simulink model "controller_sdfp_host"  (Simulink 7.3)
settings: Solver=ode45  StartTime=0.0  StopTime=2  RelTol=1e-3
values from neighbouring files (symbols this model uses):
  d = 16    [one_bit_control.m]
  fixpt_adder_in_bitwidth = w    (= 24)    [one_bit_control.m]
  fixpt_adder_in_position = d    (= 16)    [one_bit_control.m]
  fixpt_adder_out_bitwidth = w    (= 24)    [one_bit_control.m]
  fixpt_adder_out_position = d    (= 16)    [one_bit_control.m]
  fixpt_gain_bitwidth = w    (= 24)    [one_bit_control.m]
  fixpt_gain_position = d    (= 16)    [one_bit_control.m]
  k = 2^k_bitshift    (= 0.0001220703125)    [one_bit_control.m]
  p0 = (109.9*Ki)*T^3*k^-3    [one_bit_control.m]
  p1 = (20.78*Ki+109.9*Kp)*T^2*k^-2    [one_bit_control.m]
  p2 = (Ki+20.78*Kp)*T*k^-1    [one_bit_control.m]
  p3 = Kp    (= 8)    [one_bit_control.m]
  q0 = 0*T^3*k^-3    [one_bit_control.m]
  q1 = 174.8*T^2*k^-2    [one_bit_control.m]
  q2 = 26.33*T*k^-1    [one_bit_control.m]
  T = ts    [one_bit_control.m]
  ts = 1/Fs    [one_bit_control.m]
  ts_k_gain1 = k_bitshift - Fs_power_2    [one_bit_control.m]
  ts_k_gain2 = k_bitshift - Fs_power_2    [one_bit_control.m]
  ts_k_gain3 = k_bitshift - Fs_power_2    [one_bit_control.m]
  w = 24    [one_bit_control.m]
libraries: simulink x16, cstblocks x5, commnoisgen2 x1, simulink_extras x1
(part 2 of 2)

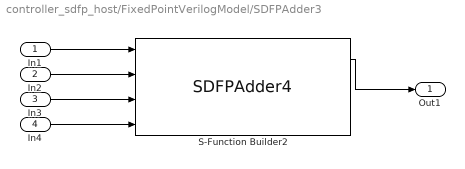
== system controller_sdfp_host/FixedPointVerilogModel/SDFPAdder3 ==
  In1 : Inport  OutDataType=fixdt(1, 16)  OutScaling=2^0
  In2 : Inport  Port=2  OutDataType=fixdt(1, 16)  OutScaling=2^0
  In3 : Inport  Port=3  OutDataType=fixdt(1, 16)  OutScaling=2^0
  In4 : Inport  Port=4  OutDataType=fixdt(1, 16)  OutScaling=2^0
  S-Function Builder2 : S-Function  InitFcn=try, set_param(gcb,'FunctionName','SDFPAdder4'), end  FunctionName=SDFPAdder4  Parameters=uint32(in_bitwidth),uint32(in_fp_position),uint32(out_bitwidth),uint32(out_fp_position)  SFunctionModules=SDFPAdder4_wrapper  WizardData=DataTag17  EnableBusSupport=off  mask(S-Function Builder){}
      mask help: The S-Function Builder block creates a wrapper C-MEX S-function from your supplied C code with multiple input ports, output ports, and a variable number of scalar, vector, or matrix parameters. The input and output ports can propagate Simulink built-in data types, fixed-point datatypes, complex, frame, 1-D, and 2-D signals. This block also supports discrete and continuous states of type real. You can optionally have the block generate a TLC file to be used with Real-Time Workshop for code generation.
      mask init: same as controller_sdfp_host/FixedPointVerilogModel/FloatForScope1/S-Function Builder
      settings: CopyFcn=set_param(gcbh,'LinkStatus','none')  PreSaveFcn=try, set_param(gcb,'FunctionName','SDFPAdder4'), end  OpenFcn=sfunctionwizard(gcbh)
      mask Display: plot(val(:,1),val(:,2)),disp(sys)port_label('input',1,'in0')port_label('input',2,'in1')port_label('input',3,'in2')port_label('input',4,'in3')port_label('output',1,'adder_out')
  Out1 : Outport  OutDataType=fixdt(1, 16)  OutScaling=2^0
  wires:
  In1/1 -> S-Function Builder2/1
  In2/1 -> S-Function Builder2/2
  In3/1 -> S-Function Builder2/3
  In4/1 -> S-Function Builder2/4
  S-Function Builder2/1 -> Out1/1

== system controller_sdfp_host/FixedPointVerilogModel/SDFPAdder4 ==
  In1 : Inport  OutDataType=fixdt(1, 16)  OutScaling=2^0
  In2 : Inport  Port=2  OutDataType=fixdt(1, 16)  OutScaling=2^0
  In3 : Inport  Port=3  OutDataType=fixdt(1, 16)  OutScaling=2^0
  In4 : Inport  Port=4  OutDataType=fixdt(1, 16)  OutScaling=2^0
  S-Function Builder2 : S-Function  InitFcn=try, set_param(gcb,'FunctionName','SDFPAdder4'), end  FunctionName=SDFPAdder4  Parameters=uint32(in_bitwidth),uint32(in_fp_position),uint32(out_bitwidth),uint32(out_fp_position)  SFunctionModules=SDFPAdder4_wrapper  WizardData=DataTag18  EnableBusSupport=off  mask(S-Function Builder){}
      mask help: The S-Function Builder block creates a wrapper C-MEX S-function from your supplied C code with multiple input ports, output ports, and a variable number of scalar, vector, or matrix parameters. The input and output ports can propagate Simulink built-in data types, fixed-point datatypes, complex, frame, 1-D, and 2-D signals. This block also supports discrete and continuous states of type real. You can optionally have the block generate a TLC file to be used with Real-Time Workshop for code generation.
      mask init: same as controller_sdfp_host/FixedPointVerilogModel/FloatForScope1/S-Function Builder
      settings: CopyFcn=set_param(gcbh,'LinkStatus','none')  PreSaveFcn=try, set_param(gcb,'FunctionName','SDFPAdder4'), end  OpenFcn=sfunctionwizard(gcbh)
      mask Display: plot(val(:,1),val(:,2)),disp(sys)port_label('input',1,'in0')port_label('input',2,'in1')port_label('input',3,'in2')port_label('input',4,'in3')port_label('output',1,'adder_out')
  Out1 : Outport  OutDataType=fixdt(1, 16)  OutScaling=2^0
  wires:
  In1/1 -> S-Function Builder2/1
  In2/1 -> S-Function Builder2/2
  In3/1 -> S-Function Builder2/3
  In4/1 -> S-Function Builder2/4
  S-Function Builder2/1 -> Out1/1

== system controller_sdfp_host/FixedPointVerilogModel/SDFPFromFixed ==
  In1 : Inport  OutDataType=fixdt(1, 16)  OutScaling=2^0
  S-Function Builder : S-Function  InitFcn=try, set_param(gcb,'FunctionName','SDFPFromFixed'), end  FunctionName=SDFPFromFixed  Parameters=uint32(bitwidth),uint32(fp_position)  SFunctionModules=SDFPFromFixed_wrapper fpconv  WizardData=DataTag19  EnableBusSupport=off  mask(S-Function Builder){}
      mask help: The S-Function Builder block creates a wrapper C-MEX S-function from your supplied C code with multiple input ports, output ports, and a variable number of scalar, vector, or matrix parameters. The input and output ports can propagate Simulink built-in data types, fixed-point datatypes, complex, frame, 1-D, and 2-D signals. This block also supports discrete and continuous states of type real. You can optionally have the block generate a TLC file to be used with Real-Time Workshop for code generation.
      mask init: same as controller_sdfp_host/FixedPointVerilogModel/FloatForScope1/S-Function Builder
      settings: CopyFcn=set_param(gcbh,'LinkStatus','none')  PreSaveFcn=try, set_param(gcb,'FunctionName','SDFPFromFixed'), end  OpenFcn=sfunctionwizard(gcbh)
      mask Display: plot(val(:,1),val(:,2)),disp(sys)port_label('input',1,'fixed_in')port_label('output',1,'float_out')
  Out1 : Outport  OutDataType=fixdt(1, 16)  OutScaling=2^0
  wires:
  In1/1 -> S-Function Builder/1
  S-Function Builder/1 -> Out1/1

== system controller_sdfp_host/FixedPointVerilogModel/SDFPShifter ==
  In1 : Inport  OutDataType=fixdt(1, 16)  OutScaling=2^0
  S-Function Builder3 : S-Function  InitFcn=try, set_param(gcb,'FunctionName','SDFPShifter'), end  FunctionName=SDFPShifter  Parameters=int32(shift_amount)  SFunctionModules=SDFPShifter_wrapper  WizardData=DataTag20  EnableBusSupport=off  mask(S-Function Builder){}
      mask help: The S-Function Builder block creates a wrapper C-MEX S-function from your supplied C code with multiple input ports, output ports, and a variable number of scalar, vector, or matrix parameters. The input and output ports can propagate Simulink built-in data types, fixed-point datatypes, complex, frame, 1-D, and 2-D signals. This block also supports discrete and continuous states of type real. You can optionally have the block generate a TLC file to be used with Real-Time Workshop for code generation.
      mask init: same as controller_sdfp_host/FixedPointVerilogModel/FloatForScope1/S-Function Builder
      settings: CopyFcn=set_param(gcbh,'LinkStatus','none')  PreSaveFcn=try, set_param(gcb,'FunctionName','SDFPShifter'), end  OpenFcn=sfunctionwizard(gcbh)
      mask Display: plot(val(:,1),val(:,2)),disp(sys)port_label('input',1,'sg_in')port_label('output',1,'shifter_out')
  Out1 : Outport  OutDataType=fixdt(1, 16)  OutScaling=2^0
  wires:
  In1/1 -> S-Function Builder3/1
  S-Function Builder3/1 -> Out1/1

== system controller_sdfp_host/FixedPointVerilogModel/SDFPToFixed ==
  In1 : Inport  OutDataType=fixdt(1, 16)  OutScaling=2^0
  S-Function Builder : S-Function  InitFcn=try, set_param(gcb,'FunctionName','SDFPToFixed'), end  FunctionName=SDFPToFixed  Parameters=uint32(bitwidth),uint32(fp_position)  SFunctionModules=SDFPToFixed_wrapper fpconv  WizardData=DataTag21  EnableBusSupport=off  mask(S-Function Builder){}
      mask help: The S-Function Builder block creates a wrapper C-MEX S-function from your supplied C code with multiple input ports, output ports, and a variable number of scalar, vector, or matrix parameters. The input and output ports can propagate Simulink built-in data types, fixed-point datatypes, complex, frame, 1-D, and 2-D signals. This block also supports discrete and continuous states of type real. You can optionally have the block generate a TLC file to be used with Real-Time Workshop for code generation.
      mask init: same as controller_sdfp_host/FixedPointVerilogModel/FloatForScope1/S-Function Builder
      settings: CopyFcn=set_param(gcbh,'LinkStatus','none')  PreSaveFcn=try, set_param(gcb,'FunctionName','SDFPToFixed'), end  OpenFcn=sfunctionwizard(gcbh)
      mask Display: plot(val(:,1),val(:,2)),disp(sys)port_label('input',1,'float_in')port_label('output',1,'fixed_out')
  Out1 : Outport  OutDataType=fixdt(1, 16)  OutScaling=2^0
  wires:
  In1/1 -> S-Function Builder/1
  S-Function Builder/1 -> Out1/1

== system controller_sdfp_host/FixedPointVerilogModel/Subsystem ==
  In1 : Inport  OutDataType=fixdt(1, 16)  OutScaling=2^0
  S-Function Builder : S-Function  InitFcn=try, set_param(gcb,'FunctionName','SDFPGainSwitch'), end  FunctionName=SDFPGainSwitch  Parameters=single(gain),uint32(bitwidth),uint32(fp_position)  SFunctionModules=SDFPGainSwitch_wrapper fpconv  WizardData=DataTag22  EnableBusSupport=off  mask(S-Function Builder){}
      mask help: The S-Function Builder block creates a wrapper C-MEX S-function from your supplied C code with multiple input ports, output ports, and a variable number of scalar, vector, or matrix parameters. The input and output ports can propagate Simulink built-in data types, fixed-point datatypes, complex, frame, 1-D, and 2-D signals. This block also supports discrete and continuous states of type real. You can optionally have the block generate a TLC file to be used with Real-Time Workshop for code generation.
      mask init: same as controller_sdfp_host/FixedPointVerilogModel/FloatForScope1/S-Function Builder
      settings: CopyFcn=set_param(gcbh,'LinkStatus','none')  PreSaveFcn=try, set_param(gcb,'FunctionName','SDFPGainSwitch'), end  OpenFcn=sfunctionwizard(gcbh)
      mask Display: plot(val(:,1),val(:,2)),disp(sys)port_label('input',1,'sd_in')port_label('output',1,'gain_out')
  Out1 : Outport  OutDataType=fixdt(1, 16)  OutScaling=2^0
  wires:
  S-Function Builder/1 -> Out1/1
  In1/1 -> S-Function Builder/1

== system controller_sdfp_host/FixedPointVerilogModel/ts_and_k_gain1 ==
  In1 : Inport  OutDataType=fixdt(1, 16)  OutScaling=2^0
  S-Function Builder3 : S-Function  InitFcn=try, set_param(gcb,'FunctionName','SDFPShifter'), end  FunctionName=SDFPShifter  Parameters=int32(shift_amount)  SFunctionModules=SDFPShifter_wrapper  WizardData=DataTag23  EnableBusSupport=off  mask(S-Function Builder){}
      mask help: The S-Function Builder block creates a wrapper C-MEX S-function from your supplied C code with multiple input ports, output ports, and a variable number of scalar, vector, or matrix parameters. The input and output ports can propagate Simulink built-in data types, fixed-point datatypes, complex, frame, 1-D, and 2-D signals. This block also supports discrete and continuous states of type real. You can optionally have the block generate a TLC file to be used with Real-Time Workshop for code generation.
      mask init: same as controller_sdfp_host/FixedPointVerilogModel/FloatForScope1/S-Function Builder
      settings: CopyFcn=set_param(gcbh,'LinkStatus','none')  PreSaveFcn=try, set_param(gcb,'FunctionName','SDFPShifter'), end  OpenFcn=sfunctionwizard(gcbh)
      mask Display: plot(val(:,1),val(:,2)),disp(sys)port_label('input',1,'sg_in')port_label('output',1,'shifter_out')
  Out1 : Outport  OutDataType=fixdt(1, 16)  OutScaling=2^0
  wires:
  In1/1 -> S-Function Builder3/1
  S-Function Builder3/1 -> Out1/1

== system controller_sdfp_host/FixedPointVerilogModel/ts_and_k_gain2 ==
  In1 : Inport  OutDataType=fixdt(1, 16)  OutScaling=2^0
  S-Function Builder3 : S-Function  InitFcn=try, set_param(gcb,'FunctionName','SDFPShifter'), end  FunctionName=SDFPShifter  Parameters=int32(shift_amount)  SFunctionModules=SDFPShifter_wrapper  WizardData=DataTag24  EnableBusSupport=off  mask(S-Function Builder){}
      mask help: The S-Function Builder block creates a wrapper C-MEX S-function from your supplied C code with multiple input ports, output ports, and a variable number of scalar, vector, or matrix parameters. The input and output ports can propagate Simulink built-in data types, fixed-point datatypes, complex, frame, 1-D, and 2-D signals. This block also supports discrete and continuous states of type real. You can optionally have the block generate a TLC file to be used with Real-Time Workshop for code generation.
      mask init: same as controller_sdfp_host/FixedPointVerilogModel/FloatForScope1/S-Function Builder
      settings: CopyFcn=set_param(gcbh,'LinkStatus','none')  PreSaveFcn=try, set_param(gcb,'FunctionName','SDFPShifter'), end  OpenFcn=sfunctionwizard(gcbh)
      mask Display: plot(val(:,1),val(:,2)),disp(sys)port_label('input',1,'sg_in')port_label('output',1,'shifter_out')
  Out1 : Outport  OutDataType=fixdt(1, 16)  OutScaling=2^0
  wires:
  S-Function Builder3/1 -> Out1/1
  In1/1 -> S-Function Builder3/1

== system controller_sdfp_host/FixedPointVerilogModel/ts_and_k_gain3 ==
  In1 : Inport  OutDataType=fixdt(1, 16)  OutScaling=2^0
  S-Function Builder3 : S-Function  InitFcn=try, set_param(gcb,'FunctionName','SDFPShifter'), end  FunctionName=SDFPShifter  Parameters=int32(shift_amount)  SFunctionModules=SDFPShifter_wrapper  WizardData=DataTag25  EnableBusSupport=off  mask(S-Function Builder){}
      mask help: The S-Function Builder block creates a wrapper C-MEX S-function from your supplied C code with multiple input ports, output ports, and a variable number of scalar, vector, or matrix parameters. The input and output ports can propagate Simulink built-in data types, fixed-point datatypes, complex, frame, 1-D, and 2-D signals. This block also supports discrete and continuous states of type real. You can optionally have the block generate a TLC file to be used with Real-Time Workshop for code generation.
      mask init: same as controller_sdfp_host/FixedPointVerilogModel/FloatForScope1/S-Function Builder
      settings: CopyFcn=set_param(gcbh,'LinkStatus','none')  PreSaveFcn=try, set_param(gcb,'FunctionName','SDFPShifter'), end  OpenFcn=sfunctionwizard(gcbh)
      mask Display: plot(val(:,1),val(:,2)),disp(sys)port_label('input',1,'sg_in')port_label('output',1,'shifter_out')
  Out1 : Outport  OutDataType=fixdt(1, 16)  OutScaling=2^0
  wires:
  In1/1 -> S-Function Builder3/1
  S-Function Builder3/1 -> Out1/1

== system controller_sdfp_host/SecondOrder Sigdel1/Compare to Zero ==
  In1 : Inport  OutDataType=sfix(16)  OutScaling=2^0
  Compare To Zero : simulink/Logic and Bit Operations/Compare To Zero  SystemSampleTime=-1  relop=>=  LogicOutDataTypeMode=uint8
  Constant : Constant  OutDataType=sfix(16)  OutScaling=2^0
  Constant1 : Constant  Value=-1  OutDataType=sfix(16)  OutScaling=2^0
  Switch : Switch  Threshold=0.5
  Out1 : Outport  OutDataType=sfix(16)  OutScaling=2^0
  wires:
  Constant1/1 -> Switch/3
  Constant/1 -> Switch/1
  Compare To Zero/1 -> Switch/2
  In1/1 -> Compare To Zero/1
  Switch/1 -> Out1/1

== system controller_sdfp_host/SecondOrder Sigdel2/Compare to Zero ==
  In1 : Inport  OutDataType=sfix(16)  OutScaling=2^0
  Compare To Zero : simulink/Logic and Bit Operations/Compare To Zero  SystemSampleTime=-1  relop=>=  LogicOutDataTypeMode=uint8
  Constant : Constant  OutDataType=sfix(16)  OutScaling=2^0
  Constant1 : Constant  Value=-1  OutDataType=sfix(16)  OutScaling=2^0
  Switch : Switch  Threshold=0.5
  Out1 : Outport  OutDataType=sfix(16)  OutScaling=2^0
  wires:
  Constant1/1 -> Switch/3
  Constant/1 -> Switch/1
  Compare To Zero/1 -> Switch/2
  In1/1 -> Compare To Zero/1
  Switch/1 -> Out1/1

== system controller_sdfp_host/SecondOrder Sigdel3/Compare to Zero ==
  In1 : Inport  OutDataType=sfix(16)  OutScaling=2^0
  Compare To Zero : simulink/Logic and Bit Operations/Compare To Zero  SystemSampleTime=-1  relop=>=  LogicOutDataTypeMode=uint8
  Constant : Constant  OutDataType=sfix(16)  OutScaling=2^0
  Constant1 : Constant  Value=-1  OutDataType=sfix(16)  OutScaling=2^0
  Switch : Switch  Threshold=0.5
  Out1 : Outport  OutDataType=sfix(16)  OutScaling=2^0
  wires:
  Constant1/1 -> Switch/3
  Constant/1 -> Switch/1
  Compare To Zero/1 -> Switch/2
  In1/1 -> Compare To Zero/1
  Switch/1 -> Out1/1

== system controller_sdfp_host/FixedPointVerilogModel/SDFPAdder1/GM1Float ==
  In1 : Inport  OutDataType=fixdt(1, 16)  OutScaling=2^0
  S-Function Builder : S-Function  InitFcn=try, set_param(gcb,'FunctionName','SDFPFromFixed'), end  FunctionName=SDFPFromFixed  Parameters=uint32(bitwidth),uint32(fp_position)  SFunctionModules=SDFPFromFixed_wrapper fpconv  WizardData=DataTag12  EnableBusSupport=off  mask(S-Function Builder){}
      mask help: The S-Function Builder block creates a wrapper C-MEX S-function from your supplied C code with multiple input ports, output ports, and a variable number of scalar, vector, or matrix parameters. The input and output ports can propagate Simulink built-in data types, fixed-point datatypes, complex, frame, 1-D, and 2-D signals. This block also supports discrete and continuous states of type real. You can optionally have the block generate a TLC file to be used with Real-Time Workshop for code generation.
      mask init: same as controller_sdfp_host/FixedPointVerilogModel/FloatForScope1/S-Function Builder
      settings: CopyFcn=set_param(gcbh,'LinkStatus','none')  PreSaveFcn=try, set_param(gcb,'FunctionName','SDFPFromFixed'), end  OpenFcn=sfunctionwizard(gcbh)
      mask Display: plot(val(:,1),val(:,2)),disp(sys)port_label('input',1,'fixed_in')port_label('output',1,'float_out')
  Out1 : Outport  OutDataType=fixdt(1, 16)  OutScaling=2^0
  wires:
  In1/1 -> S-Function Builder/1
  S-Function Builder/1 -> Out1/1

== system controller_sdfp_host/FixedPointVerilogModel/SDFPAdder1/GM1Float1 ==
  In1 : Inport  OutDataType=fixdt(1, 16)  OutScaling=2^0
  S-Function Builder : S-Function  InitFcn=try, set_param(gcb,'FunctionName','SDFPFromFixed'), end  FunctionName=SDFPFromFixed  Parameters=uint32(bitwidth),uint32(fp_position)  SFunctionModules=SDFPFromFixed_wrapper fpconv  WizardData=DataTag13  EnableBusSupport=off  mask(S-Function Builder){}
      mask help: The S-Function Builder block creates a wrapper C-MEX S-function from your supplied C code with multiple input ports, output ports, and a variable number of scalar, vector, or matrix parameters. The input and output ports can propagate Simulink built-in data types, fixed-point datatypes, complex, frame, 1-D, and 2-D signals. This block also supports discrete and continuous states of type real. You can optionally have the block generate a TLC file to be used with Real-Time Workshop for code generation.
      mask init: same as controller_sdfp_host/FixedPointVerilogModel/FloatForScope1/S-Function Builder
      settings: CopyFcn=set_param(gcbh,'LinkStatus','none')  PreSaveFcn=try, set_param(gcb,'FunctionName','SDFPFromFixed'), end  OpenFcn=sfunctionwizard(gcbh)
      mask Display: plot(val(:,1),val(:,2)),disp(sys)port_label('input',1,'fixed_in')port_label('output',1,'float_out')
  Out1 : Outport  OutDataType=fixdt(1, 16)  OutScaling=2^0
  wires:
  In1/1 -> S-Function Builder/1
  S-Function Builder/1 -> Out1/1

== system controller_sdfp_host/FixedPointVerilogModel/SDFPAdder1/GM1Float2 ==
  In1 : Inport  OutDataType=fixdt(1, 16)  OutScaling=2^0
  S-Function Builder : S-Function  InitFcn=try, set_param(gcb,'FunctionName','SDFPFromFixed'), end  FunctionName=SDFPFromFixed  Parameters=uint32(bitwidth),uint32(fp_position)  SFunctionModules=SDFPFromFixed_wrapper fpconv  WizardData=DataTag14  EnableBusSupport=off  mask(S-Function Builder){}
      mask help: The S-Function Builder block creates a wrapper C-MEX S-function from your supplied C code with multiple input ports, output ports, and a variable number of scalar, vector, or matrix parameters. The input and output ports can propagate Simulink built-in data types, fixed-point datatypes, complex, frame, 1-D, and 2-D signals. This block also supports discrete and continuous states of type real. You can optionally have the block generate a TLC file to be used with Real-Time Workshop for code generation.
      mask init: same as controller_sdfp_host/FixedPointVerilogModel/FloatForScope1/S-Function Builder
      settings: CopyFcn=set_param(gcbh,'LinkStatus','none')  PreSaveFcn=try, set_param(gcb,'FunctionName','SDFPFromFixed'), end  OpenFcn=sfunctionwizard(gcbh)
      mask Display: plot(val(:,1),val(:,2)),disp(sys)port_label('input',1,'fixed_in')port_label('output',1,'float_out')
  Out1 : Outport  OutDataType=fixdt(1, 16)  OutScaling=2^0
  wires:
  In1/1 -> S-Function Builder/1
  S-Function Builder/1 -> Out1/1
